simulink model "simlab2"  (R2020b)
settings: Solver=FixedStepAuto  StartTime=0.0  StopTime=40.0  FixedStep=0.01  RelTol=1e-3
values from neighbouring files (symbols this model uses):
  A = 1    [lab2.m]
  k = 1    [lab2.m]
  T = 1    [lab2.m]
  tau = 3    [lab2.m]
  w0 = 1.38    [lab2.m]
  w1 = 0.61    [lab2.m]
libraries: simulink x4
settings Model: Creator=wojciechkonury  LastModifiedBy=pkubo

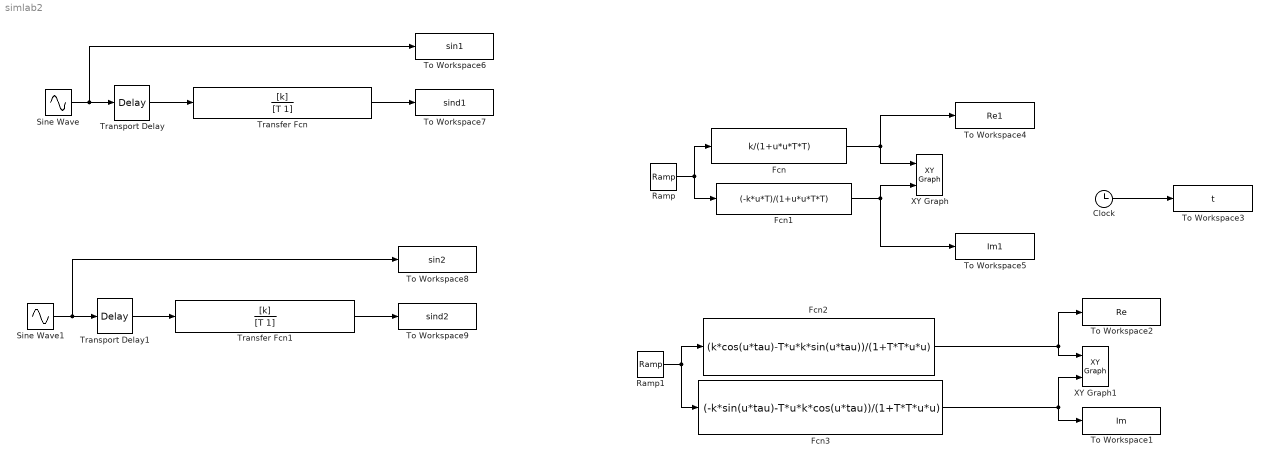
== system simlab2 ==
  Clock : Clock
  Fcn : Fcn  Expr=k/(1+u*u*T*T)
  Fcn1 : Fcn  Expr=(-k*u*T)/(1+u*u*T*T)
  Fcn2 : Fcn  Expr=(k*cos(u*tau)-T*u*k*sin(u*tau))/(1+T*T*u*u)
  Fcn3 : Fcn  Expr=(-k*sin(u*tau)-T*u*k*cos(u*tau))/(1+T*T*u*u)
  Ramp : simulink/Sources/Ramp  slope=1  start=0  InitialOutput=0
  Ramp1 : simulink/Sources/Ramp  slope=1  start=0  InitialOutput=0
  Sine Wave : Sin  Amplitude=A  Frequency=w0  SampleTime=0
  Sine Wave1 : Sin  Frequency=w1  SampleTime=0
  To Workspace1 : ToWorkspace  VariableName=Im  SampleTime=-1
  To Workspace2 : ToWorkspace  VariableName=Re  SampleTime=-1
  To Workspace3 : ToWorkspace  VariableName=t  SampleTime=-1
  To Workspace4 : ToWorkspace  VariableName=Re1  SampleTime=-1
  To Workspace5 : ToWorkspace  VariableName=Im1  SampleTime=-1
  To Workspace6 : ToWorkspace  VariableName=sin1  SampleTime=-1
  To Workspace7 : ToWorkspace  VariableName=sind1  SampleTime=-1
  To Workspace8 : ToWorkspace  VariableName=sin2  SampleTime=-1
  To Workspace9 : ToWorkspace  VariableName=sind2  SampleTime=-1
  Transfer Fcn : TransferFcn  Numerator=[k]  Denominator=[T 1]
  Transfer Fcn1 : TransferFcn  Numerator=[k]  Denominator=[T 1]
  Transport Delay : TransportDelay  DelayTime=tau  FixedBuffer=on
  Transport Delay1 : TransportDelay  DelayTime=tau  FixedBuffer=on
  XY Graph : simulink/Sinks/XY Graph  xmin=-1  xmax=1  ymin=-1  ymax=1  st=-1
  XY Graph1 : simulink/Sinks/XY Graph  xmin=-1  xmax=1  ymin=-1  ymax=1  st=-1
  wires:
  Ramp/1 -> Fcn1/1, Fcn/1
  Fcn1/1 -> To Workspace5/1, XY Graph/2
  Fcn/1 -> To Workspace4/1, XY Graph/1
  Fcn2/1 -> To Workspace2/1, XY Graph1/1
  Ramp1/1 -> Fcn3/1, Fcn2/1
  Fcn3/1 -> XY Graph1/2, To Workspace1/1
  Clock/1 -> To Workspace3/1
  Sine Wave/1 -> To Workspace6/1, Transport Delay/1
  Transport Delay/1 -> Transfer Fcn/1
  Transfer Fcn/1 -> To Workspace7/1
  Sine Wave1/1 -> To Workspace8/1, Transport Delay1/1
  Transport Delay1/1 -> Transfer Fcn1/1
  Transfer Fcn1/1 -> To Workspace9/1
